simulink model "classification_model_1"  (R2018b)
settings: Solver=daessc  StartTime=0.0  StopTime=1  RelTol=1e-3
StopFcn:
  | fault_type = 1005;
  | location = 50;
  | current = c(:,2:4);
  | current(:,4) = fault_type;
  | current(:,5) = location;
  | voltage = v(:,2:4);
  | logg = [voltage,current];
  | data = xlsread('sdata1');
  | data = [data;logg];
  | xlswrite('sdata1',data);
libraries: powerlib x7, powerlib_meascontrol x2
settings Model: Creator=Edagotti Pavankumar  LastModifiedBy=Edagotti Pavankumar
settings SolverCC: ZeroCrossAlgorithm=Adaptive
settings DebuggingCC: IgnoredZcDiagnostic=none

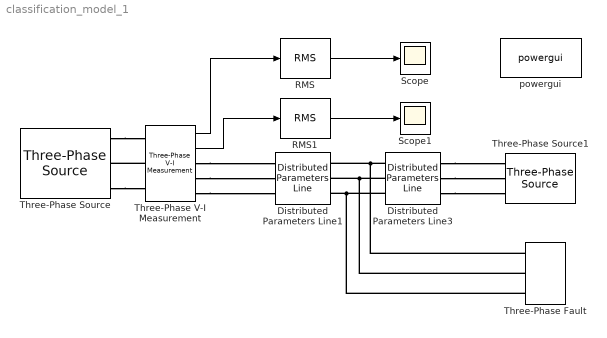
== system classification_model_1 ==
  Distributed Parameters Line1 : powerlib/Elements/Distributed Parameters Line  Phases=3  Frequency=50  Resistance=[0.0238 0.3885]  Inductance=[0.0009509508 0.0032508989]  Capacitance=[12.74e-9 7.751e-9]  Length=50  x1=[2.47382558882236e-10 272937.603824643 272937.603824645;314.159265358979 314.159265358979 314.159265358979;1.49194654837244 0.434043679615576 -1.13675264717932]  x2=[2.99995417707953e-10 274167.064757833 274167.064757835;314.159265358979 314.159265358979 314.159265358979;1.7369252114993 0.433676655897655 -1.13711967089724]  x3=[2.63915937924335e-12 1001.56472405765 1001.56472405766;314.159265358979 314.159265358979 314.159265358979;0.638982217538489 0.324556739532947 -1.24623958726195]  x4=[1.31712686807063e-12 1001.88717060074 1001.88717060074;314.159265358979 314.159265358979 314.159265358979;3.10527040978712 0.488402443149096 -1.08239388364581]  x5=0.000250986639952707  V1=[2.474e-10 2.729e+05 2.729e+05;314.2 314.2 314.2;1.492 0.434 -1.137]  V2=[3e-10 2.742e+05 2.742e+05;314.2 314.2 314.2;1.737 0.4337 -1.137]  I1=[2.639e-12 1002 1002;314.2 314.2 314.2;0.639 0.3246 -1.246]  I2=[1.317e-12 1002 1002;314.2 314.2 314.2;3.105 0.4884 -1.082]  nHarmo=1  Measurements=None
      settings: SourceProductName=Simscape Power Systems
  Distributed Parameters Line3 : powerlib/Elements/Distributed Parameters Line  Phases=3  Frequency=50  Resistance=[0.0238 0.3885]  Inductance=[0.0009509508 0.0032508989]  Capacitance=[12.74e-9 7.751e-9]  Length=150  x1=[2.99995417707953e-10 274167.064757833 274167.064757835;314.159265358979 314.159265358979 314.159265358979;1.57922565465438 0.324327959298446 -1.24646836749645]  x2=[2.31119049920651e-10 272937.917712324 272937.917712326;314.159265358979 314.159265358979 314.159265358979;1.82605616751621 0.324708516630805 -1.24608781016409]  x3=[3.16866873925465e-13 995.345525673914 995.345525673921;314.159265358979 314.159265358979 314.159265358979;2.36462381805183 0.269481792955061 -1.30131453383984]  x4=[1.02712547190807e-12 995.079620101289 995.079620101293;314.159265358979 314.159265358979 314.159265358979;1.98832971594187 0.214986476792083 -1.35580985000282]  x5=0.000752959919858122  V1=[3e-10 2.742e+05 2.742e+05;314.2 314.2 314.2;1.579 0.3243 -1.246]  V2=[2.311e-10 2.729e+05 2.729e+05;314.2 314.2 314.2;1.826 0.3247 -1.246]  I1=[3.169e-13 995.3 995.3;314.2 314.2 314.2;2.365 0.2695 -1.301]  I2=[1.027e-12 995.1 995.1;314.2 314.2 314.2;1.988 0.215 -1.356]  nHarmo=1  Measurements=None
      settings: SourceProductName=Simscape Power Systems
  RMS : powerlib_meascontrol/Measurements/RMS  TrueRMS=on  Freq=50  RMSInit=0  Ts=0
  RMS1 : powerlib_meascontrol/Measurements/RMS  TrueRMS=on  Freq=50  RMSInit=0  Ts=0
  Scope : Scope
  Scope1 : Scope
  Three-Phase V-I Measurement : powerlib/Measurements/Three-Phase V-I Measurement  VoltageMeasurement=phase-to-ground  SetLabelV=off  LabelV=Vabc  Vpu=on  VpuLL=off  CurrentMeasurement=yes  SetLabelI=off  LabelI=Iabc  Ipu=on  Pbase=100e6  Vbase=220e3  OutputType=Complex  PhasorSimulation=off  PSBequivalent=0
  Three-Phase Fault : powerlib/Elements/Three-Phase Fault  InitialStates=0  FaultA=off  FaultB=on  FaultC=on  GroundFault=off  SwitchTimes=0.5  External=off  SwitchStatus=NaN  FaultResistance=20  GroundResistance=0.001  SnubberResistance=1e6  SnubberCapacitance=inf  Measurements=None
  Three-Phase Source : powerlib/Electrical Sources/Three-Phase Source  InternalConnection=Yg  VoltagePhases=off  Voltage=220e3  PhaseAngle=0  Voltage_phases=[25e3 25e3 25e3]/sqrt(3)  PhaseAngles_phases=[0 -120 +120]  Frequency=50  NonIdealSource=on  SpecifyImpedance=on  Resistance=0.8929  Inductance=16.58e-3  ShortCircuitLevel=100e6  BaseVoltage=220e3  XRratio=7  BusType=swing  Pref=10e3  Qref=0  Prefabc=[10e3, 10e3, 10e3]  Qrefabc=[0, 0, 0]  Qmin=-inf  Qmax=inf
  Three-Phase Source1 : powerlib/Electrical Sources/Three-Phase Source  InternalConnection=Yg  VoltagePhases=off  Voltage=220e3  PhaseAngle=0  Voltage_phases=[25e3 25e3 25e3]/sqrt(3)  PhaseAngles_phases=[0 -120 +120]  Frequency=50  NonIdealSource=on  SpecifyImpedance=on  Resistance=0.8929  Inductance=16.58e-3  ShortCircuitLevel=100e6  BaseVoltage=220e3  XRratio=7  BusType=PV  Pref=inf  Qref=0  Prefabc=[10e3, 10e3, 10e3]  Qrefabc=[0, 0, 0]  Qmin=-inf  Qmax=inf
  powergui : powerlib/powergui  Priority=1  SimulationMode=Continuous  SampleTime=50e-10  frequency=60  Iterations=50  frequencyindice=50  Pbase=100e6  ErrMax=1e-4  UnitsV=kV  UnitsW=MW  buscounter=0  FunctionMessages=off  echomessages=off  EnableUseOfTLC=off  CurrentSourceSwitches=off  DisableSnubberDevices=off  DisableRonSwitches=off  DisableVfSwitches=off  DisplayEquations=off  SolverType=Tustin/Backward Euler (TBE)  Interpol=off  ExternalGateDelay=off  methode=off  Ts=100  x0status=blocks  SPID=off  SwTol=0  HookPort=off  RestoreLinks=warning  ResistiveCurrentMeasurement=off  Frange=[0:2:500]  Ylog=off  Xlog=on  ShowGrid=off  save=off  variable=ZData  structure=0  ZoomFFT=off  StartTime=0.0  cycles=1  DisplayStyle=1  fundamental=60  FreqAxis=off  MaxFrequency=1000  frequencyindicesteady=1  RmsSteady=2  display=off
  wires:
  Three-Phase V-I Measurement/1 -> RMS/1
  RMS/1 -> Scope/1
  RMS1/1 -> Scope1/1
  Three-Phase V-I Measurement/2 -> RMS1/1
  connections:
  Three-Phase V-I Measurement/LConn2 -- Three-Phase Source/RConn2
  Three-Phase Source/RConn1 -- Three-Phase V-I Measurement/LConn1
  Three-Phase Source/RConn3 -- Three-Phase V-I Measurement/LConn3
  Three-Phase V-I Measurement/RConn1 -- Distributed Parameters Line1/LConn1
  Three-Phase V-I Measurement/RConn2 -- Distributed Parameters Line1/LConn2
  Three-Phase V-I Measurement/RConn3 -- Distributed Parameters Line1/LConn3
  Distributed Parameters Line3/RConn1 -- Three-Phase Source1/RConn1
  Distributed Parameters Line3/RConn2 -- Three-Phase Source1/RConn2
  Distributed Parameters Line3/RConn3 -- Three-Phase Source1/RConn3
  Distributed Parameters Line3/LConn1 -- Three-Phase Fault/LConn1 -- Distributed Parameters Line1/RConn1
  Distributed Parameters Line3/LConn2 -- Three-Phase Fault/LConn2 -- Distributed Parameters Line1/RConn2
  Distributed Parameters Line3/LConn3 -- Three-Phase Fault/LConn3 -- Distributed Parameters Line1/RConn3
